simulink model "GPCA_System_Monitor"  (Simulink 8.7)
settings: Solver=VariableStepAuto  StartTime=0.0  StopTime=10.0  RelTol=1e-3
settings Model: Creator=bourbouh  LastModifiedBy=bourbouh
settings DataIOCC: LimitDataPoints=off  SaveFormat=Dataset
settings DebuggingCC: UnderspecifiedInitializationDetection=Simplified  MergeDetectMultiDrivingBlocksExec=error
settings HardwareCC: ProdBitPerPointer=64  ProdLargestAtomicFloat=Float  ProdIntDivRoundTo=Zero  ProdEndianess=LittleEndian  ProdWordSize=64  ProdHWDeviceType=Intel->x86-64 (Windows64)
settings ModelReferenceCC: PropagateSignalLabelsOutOfModel=on
settings ConfigComp: CovModelRefEnable=off

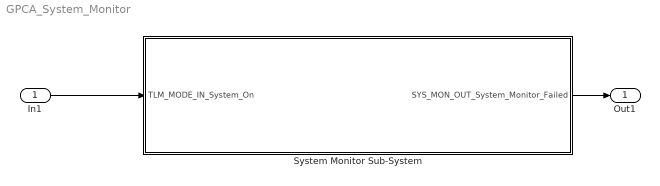
== system GPCA_System_Monitor ==
  In1 : Inport
  System Monitor Sub-System : Stateflow chart  TreatAsAtomicUnit=on
  Out1 : Outport
  wires:
  In1/1 -> System Monitor Sub-System/1(TLM_MODE_IN_System_On)
  System Monitor Sub-System/1(SYS_MON_OUT_System_Monitor_Failed) -> Out1/1

== stateflow chart System Monitor Sub-System ==
  state System_Monitor
    entry: SYS_MON_OUT_System_Monitor_Failed=0;
    during: SYS_MON_OUT_System_Monitor_Failed=0;
    exit: SYS_MON_OUT_System_Monitor_Failed=0;
  state NOT_ON
  (default) -> System_Monitor [order 1] : [TLM_MODE_IN_System_On]
  (default) -> NOT_ON [order 2]
  NOT_ON -> System_Monitor : [TLM_MODE_IN_System_On]
  System_Monitor -> NOT_ON : [!TLM_MODE_IN_System_On]
  data: TLM_MODE_IN_System_On input boolean; SYS_MON_OUT_System_Monitor_Failed output boolean
